simulink model "lab04_zad1"  (R2018a)
settings: Solver=ode4  StartTime=0.0  StopTime=100  FixedStep=2^-5  RelTol=1e-3
libraries: simulink x2
settings Model: Creator=Koala  LastModifiedBy=Koala

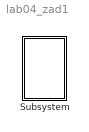
== system lab04_zad1 ==
  Subsystem : Subsystem  mask{g=9.81, l=2, m=2, k=5, r0=3, r1=1, fi0=0.1, fi1=0.1}

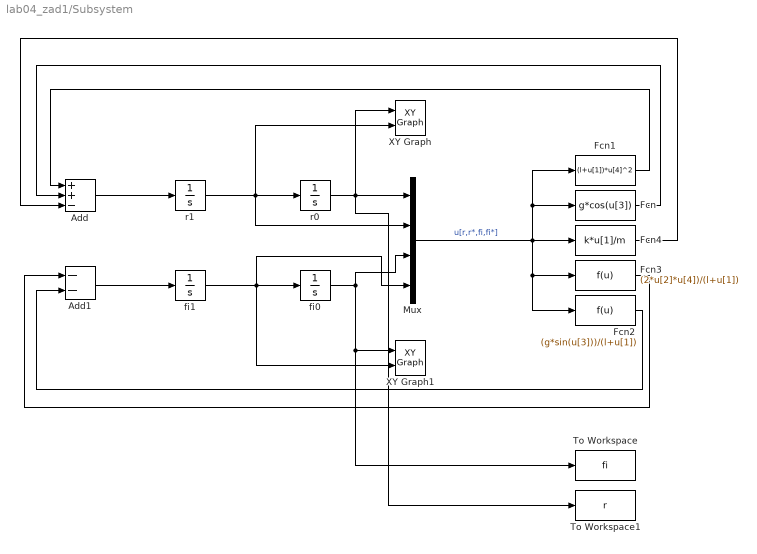
== system lab04_zad1/Subsystem ==
  Add : Sum  Inputs=++-
  Add1 : Sum  Inputs=--
  Fcn : Fcn  Expr=g*cos(u[3])
  Fcn1 : Fcn  Expr=(l+u[1])*u[4]^2
  Fcn2 : Fcn  Expr=(g*sin(u[3]))/(l+u[1])
  Fcn3 : Fcn  Expr=(2*u[2]*u[4])/(l+u[1])
  Fcn4 : Fcn  Expr=k*u[1]/m
  Mux : Mux
  To Workspace : ToWorkspace  VariableName=fi  SampleTime=-1
  To Workspace1 : ToWorkspace  VariableName=r  SampleTime=-1
  XY Graph : simulink/Sinks/XY Graph  xmin=2.5  xmax=5.5  ymin=-2  ymax=2  st=-1
  XY Graph1 : simulink/Sinks/XY Graph  xmin=-0.2  xmax=0.2  ymin=-0.2  ymax=0.2  st=-1
  fi0 : Integrator  InitialCondition=fi0
  fi1 : Integrator  InitialCondition=fi1
  r0 : Integrator  InitialCondition=r0
  r1 : Integrator  InitialCondition=r1
  wires:
  Add1/1 -> fi1/1
  Mux/1 -> Fcn3/1, Fcn2/1, Fcn/1, Fcn1/1, Fcn4/1  "u[r,r*,fi,fi*]"
  r1/1 -> XY Graph/2, Mux/2, r0/1
  Fcn3/1 -> Add1/1
  fi0/1 -> To Workspace/1, XY Graph1/1, Mux/3
  Fcn/1 -> Add/2
  Fcn2/1 -> Add1/2
  r0/1 -> To Workspace1/1, XY Graph/1, Mux/1
  Fcn1/1 -> Add/1
  fi1/1 -> Mux/4, XY Graph1/2, fi0/1
  Fcn4/1 -> Add/3
  Add/1 -> r1/1
